simulink model "problem8_stateflow"  (R2020a)
settings: Solver=FixedStepDiscrete  StartTime=0.0  StopTime=10.0  FixedStep=0.1  RelTol=1e-3  EnableMultiTasking=on
settings Model: Creator=DELL  LastModifiedBy=DELL
settings SolverCC: AutoInsertRateTranBlk=on
settings DataIOCC: LimitDataPoints=on
settings OptimizationCC: LifeSpan=inf
settings DebuggingCC: AllowSymbolicDim=off  SFUnexpectedBacktrackingDiag=warning  SFNoUnconditionalDefaultTransitionDiag=warning  SFExecutionAtInitializationDiag=none  ArithmeticOperatorsInVariantConditions=warning
settings SFSimCC: SimUseLocalCustomCode=off  CustomCodeUndefinedFunction=UseInterfaceOnly
settings RTWCC: RTWUseLocalCustomCode=off
settings CodeAppCC: StateflowObjectComments=on
settings GRTTargetCC: TargetLangStandard=C89/C90 (ANSI)
settings ConfigComp: CovMetricSettings=dw  CovHtmlReporting=on  CovSaveCumulativeToWorkspaceVar=on  CovSaveSingleToWorkspaceVar=on  CovShowResultsExplorer=off  CovExternalEMLEnable=off  CovSFcnEnable=off

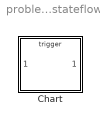
== system problem8_stateflow ==
  Chart : Stateflow chart  TreatAsAtomicUnit=on

== stateflow chart problem8_stateflow/Chart ==
  state Idle
  state PrepareLift
    entry:
    door_close = 1;
  state Active
    state LiftAction [parallel]
      settings: executionOrder=1
      state Floor_1
        entry:
        current_floor = 1;
        (default) -> (junction 47)
        (junction 47) -> (junction 57) [order 1] : [current_floor == floor_input]
        (junction 47) -> (junction 71) [order 2]
        (junction 57) -> (junction 36) : {door_close = 0;}/{Delay.count}
        (junction 36) -> (junction 71)
        (junction 71) -> (junction 58)
      state Floor_2
        entry:
        current_floor = 2;
        (default) -> (junction 52)
        (junction 52) -> (junction 69) [order 1] : [current_floor == floor_input]
        (junction 52) -> (junction 53) [order 2]
        (junction 69) -> (junction 82) : {door_close = 0;}/{Delay.count}
        (junction 82) -> (junction 53)
        (junction 53) -> (junction 59)
      state Floor_3
        entry:
        current_floor = 3;
        (default) -> (junction 74)
        (junction 74) -> (junction 66) [order 1] : [current_floor == floor_input]
        (junction 74) -> (junction 78) [order 2]
        (junction 66) -> (junction 43) : {door_close = 0;}/{Delay.count}
        (junction 43) -> (junction 78)
        (junction 78) -> (junction 38)
      state Floor_4
        entry:
        current_floor = 4;
        (default) -> (junction 37)
        (junction 37) -> (junction 83) [order 1] : [current_floor == floor_input]
        (junction 37) -> (junction 73) [order 2]
        (junction 83) -> (junction 84) : {door_close = 0;}/{Delay.count}
        (junction 84) -> (junction 73)
        (junction 73) -> (junction 31)
      state Floor_5
        entry:
        current_floor = 5;
        (default) -> (junction 17)
        (junction 17) -> (junction 18) [order 1] : [current_floor == floor_input]
        (junction 17) -> (junction 19) [order 2]
        (junction 18) -> (junction 20) : {door_close = 0;}/{Delay.count}
        (junction 20) -> (junction 19)
        (junction 19) -> (junction 21)
      (default) -> Floor_1
      Floor_1 -> Floor_2 : [floor_input>current_floor]
      Floor_2 -> Floor_1 [order 2] : [floor_input<current_floor]
      Floor_2 -> Floor_3 [order 1] : [floor_input>current_floor]
      Floor_3 -> Floor_2 [order 2] : [floor_input<current_floor]
      Floor_3 -> Floor_4 [order 1] : [floor_input>current_floor]
      Floor_4 -> Floor_3 [order 2] : [floor_input<current_floor]
      Floor_4 -> Floor_5 [order 1] : [floor_input>current_floor]
      Floor_5 -> Floor_4 : [floor_input<current_floor]
    state Delay [parallel]
      settings: executionOrder=2
      state Init
        en: i = 0;
      state Wait
        du:
        i = i+1;
      (default) -> Init
      Wait -> Init : [i>=5]{door_close=1;}
      Init -> Wait : count
  (default) -> Idle
  Active -> Idle : [door_close==1 && current_floor == floor_input]
  Idle -> PrepareLift : request
  PrepareLift -> Active
  data: floor_input input; current_floor output; door_close local; i local
  events: count local FUNCTION_CALL_EVENT; request input RISING_EDGE_EVENT
